simulink subsystem "ME_Colision"  (R2024b)
settings: Solver=VariableStepAuto  StartTime=0.0  StopTime=10.0  RelTol=1e-3
settings Model: Creator=Chenfu  LastModifiedBy=lucia

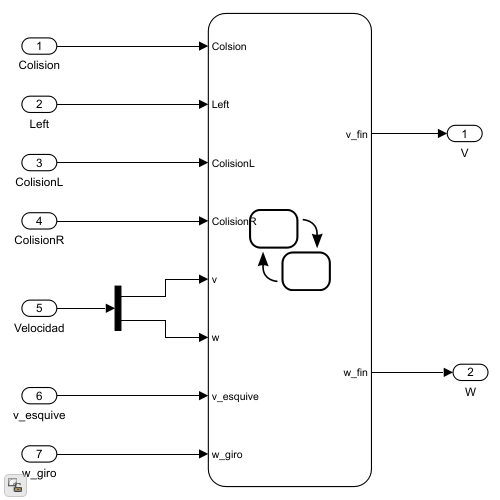
[thumbnail: Simulink's stored preview of the top-level diagram]
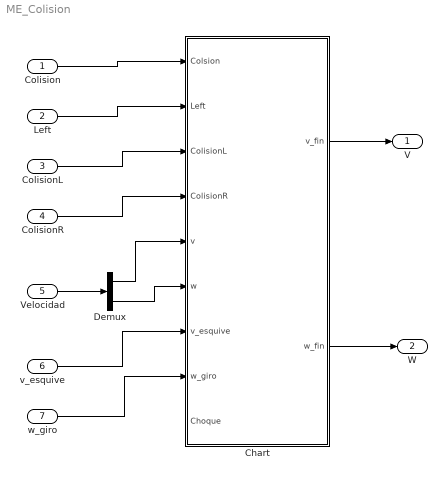
== system ME_Colision ==
  Colision : Inport
  Left : Inport  Port=2
  ColisionL : Inport  Port=3
  ColisionR : Inport  Port=4
  Velocidad : Inport  Port=5
  v_esquive : Inport  Port=6
  w_giro : Inport  Port=7
  Chart : Stateflow chart  TreatAsAtomicUnit=on
  Demux : Demux  Outputs=2
  V : Outport
  W : Outport  Port=2
  wires:
  Colision/1 -> Chart/1(Colsion)
  Chart/2(w_fin) -> W/1
  Chart/1(v_fin) -> V/1
  w_giro/1 -> Chart/8(w_giro)
  v_esquive/1 -> Chart/7(v_esquive)
  Demux/1 -> Chart/5(v)
  Demux/2 -> Chart/6(w)
  Velocidad/1 -> Demux/1
  ColisionR/1 -> Chart/4(ColisionR)
  ColisionL/1 -> Chart/3(ColisionL)
  Left/1 -> Chart/2(Left)

== stateflow chart ME_Colision/Chart ==
  state GiroDerecha
    entry:
    v_fin = 0;
    w_fin = w_giro;
  state AlejarIzquierda
    entry:
    v_fin = v_esquive;
    w_fin = -w_giro;
  state Inicializacion
    entry:
    v_fin = v;
    w_fin = w;
  state AlejarDerecha
    entry:
    v_fin = v_esquive;
    w_fin = w_giro;
  state GiroIzquierda
    entry:
    v_fin = 0;
    w_fin = -w_giro;
  AlejarIzquierda -> Inicializacion [order 2] : [Choque == 0 && ColisionR == 0]
  Inicializacion -> GiroDerecha [order 2] : [Choque == 1 && Left == 0]
  GiroDerecha -> Inicializacion [order 1] : [Choque == 0 && ColisionR == 0]
  GiroDerecha -> AlejarIzquierda [order 2] : [Choque == 0 && ColisionR == 1]
  AlejarIzquierda -> GiroDerecha [order 1] : [Choque == 1]
  Inicializacion -> AlejarIzquierda [order 4] : [Choque == 0 && ColisionR == 1]
  (default) -> Inicializacion
  Inicializacion -> AlejarDerecha [order 3] : [Choque == 0 && ColisionL == 1]
  AlejarDerecha -> Inicializacion [order 2] : [Choque == 0 && ColisionL == 0]
  Inicializacion -> GiroIzquierda [order 1] : [Choque == 1 && Left == 1]
  GiroIzquierda -> Inicializacion [order 1] : [Choque == 0 && ColisionL == 0]
  GiroIzquierda -> AlejarDerecha [order 2] : [Choque == 0 && ColisionL == 1]
  AlejarDerecha -> GiroIzquierda [order 1] : [Choque == 1]
  data: Colsion input; Left input; ColisionL input; ColisionR input; v input; w input; v_esquive input; w_giro input; v_fin output; w_fin output; Choque input
